simulink model "sl_subsys_fcncallerr2"  (Simulink 6.0)
settings: Solver=FixedStepDiscrete  StartTime=0.0  StopTime=10.0  FixedStep=1  RelTol=1e-3
settings Model: CovMetricSettings=d  Creator=The MathWorks Inc.  LastModifiedBy=batserve  ExtModeAutoUpdateStatusClock=off
settings DataIOCC: SignalLoggingName=logsOut
settings OptimizationCC: BlockReduction=off  BooleanDataType=off
settings DebuggingCC: CheckExecutionContextPreStartOutputMsg=on  CheckExecutionContextRuntimeOutputMsg=on  SolverPrmCheckMsg=none
settings HardwareCC: TargetUnknown=on

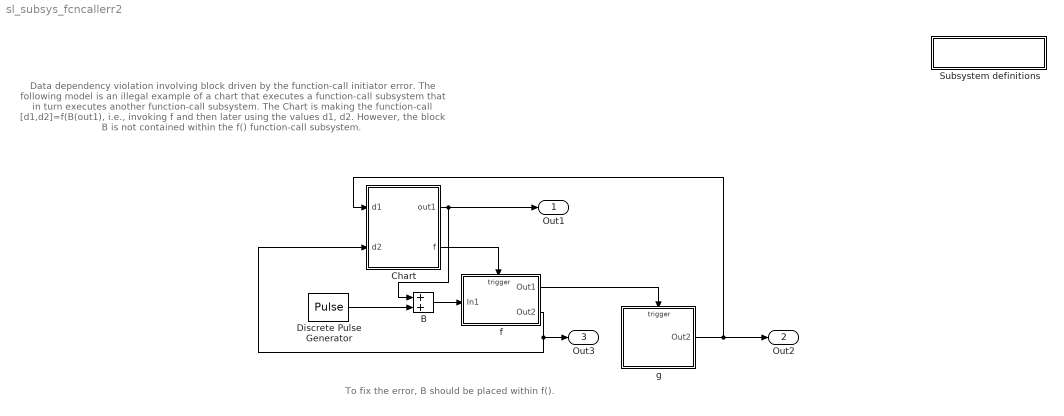
== system sl_subsys_fcncallerr2 ==
  note: Data dependency violation involving block driven by the function-call initiator error.
      |
      | The following model is an illegal example of a chart that executes a function-call
      | subsystem that in turn executes another function-call subsystem. The Chart is making
      | the function-call [d1,d2]=f(B(out1), i.e., invoking f and then later using the values
      | d1, d2. However, the block B is not contained within the f() function-call subsystem.
  note: To fix the error, B should be placed within f().
  " Subsystem definitions" : Subsystem  PropExecContextAcrossSSBoundary=on
      settings: OpenFcn=helpview([matlabroot,'/toolbox/simulink/simdemos/sl_subsys_definitions.html']);
      mask Display: disp('Subsystem\ndefinitions')
  B : Sum  SaturateOnIntegerOverflow=on  InputSameDT=on
  Chart : Stateflow chart  PropExecContextAcrossSSBoundary=on
  Discrete Pulse Generator : DiscretePulseGenerator
  f : Subsystem  TreatAsAtomicUnit=on  PropExecContextAcrossSSBoundary=on
  g : Subsystem  TreatAsAtomicUnit=on  PropExecContextAcrossSSBoundary=on
  Out1 : Outport
  Out2 : Outport  Port=2
  Out3 : Outport  Port=3
  wires:
  Chart/2(f) -> f/Trigger
  f/1(Out1) -> g/Trigger
  f/2(Out2) -> Out3/1, Chart/2(d2)
  g/1(Out2) -> Out2/1, Chart/1(d1)
  Chart/1(out1) -> Out1/1, B/1
  Discrete Pulse Generator/1 -> B/2
  B/1 -> f/1(In1)

== system sl_subsys_fcncallerr2/ Subsystem definitions ==

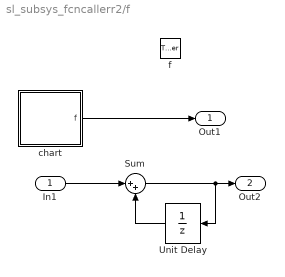
== system sl_subsys_fcncallerr2/f ==
  In1 : Inport  Port=1  LatchInput=off
  f : TriggerPort  TriggerType=function-call  StatesWhenEnabling=reset
  Sum : Sum  Inputs=|++  SaturateOnIntegerOverflow=on  InputSameDT=on
  Unit Delay : UnitDelay  Orientation=left  SampleTime=-1
  chart : Stateflow chart  PropExecContextAcrossSSBoundary=on
  Out1 : Outport
  Out2 : Outport  Port=2
  wires:
  chart/1(f) -> Out1/1
  In1/1 -> Sum/1
  Unit Delay/1 -> Sum/2
  Sum/1 -> Out2/1, Unit Delay/1

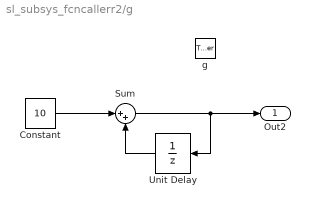
== system sl_subsys_fcncallerr2/g ==
  g : TriggerPort  TriggerType=function-call  StatesWhenEnabling=reset
  Constant : Constant  Value=10
  Sum : Sum  Inputs=|++  SaturateOnIntegerOverflow=on  InputSameDT=on
  Unit Delay : UnitDelay  Orientation=left  SampleTime=-1
  Out2 : Outport
  wires:
  Constant/1 -> Sum/1
  Unit Delay/1 -> Sum/2
  Sum/1 -> Out2/1, Unit Delay/1

== stateflow chart Chart ==
  state one/
    entry:f;out1=d1+d2;
  state two/
    entry: f;out1=d1-d2;
  one -> two
  two -> one
  (default) -> one
  data: d1 input double; d2 input double; out1 output double; out local double
  events: f output FUNCTION_CALL_EVENT

== stateflow chart f/chart ==
  state one/
    entry: f;
  state two/
    entry: f;
  one -> two
  two -> one
  (default) -> one
  events: f output FUNCTION_CALL_EVENT
